simulink model "complex_bouncing"  (Simulink 9.2)
settings: Solver=VariableStepAuto  StartTime=0.0  StopTime=5  FixedStep=1e-3  MaxStep=1e-3  RelTol=1e-6
libraries: simulink x1
settings Model: Creator=jinwooro  LastModifiedBy=jinwooro
settings SolverCC: ZeroCrossAlgorithm=Adaptive
settings DataIOCC: LimitDataPoints=off  SaveFormat=Dataset  SignalLoggingSaveFormat=Dataset
settings OptimizationCC: LifeSpan=auto
settings DebuggingCC: UnderspecifiedInitializationDetection=Simplified  MergeDetectMultiDrivingBlocksExec=error  IgnoredZcDiagnostic=none  FcnCallInpInsideContextMsg=error  StateNameClashWarn=none  SFUnexpectedBacktrackingDiag=error  SFNoUnconditionalDefaultTransitionDiag=error  SFExecutionAtInitializationDiag=warning
settings HardwareCC: ProdBitPerPointer=64  ProdBitPerSizeT=64  ProdBitPerPtrDiffT=64  ProdLargestAtomicFloat=Float  ProdIntDivRoundTo=Zero  ProdEndianess=LittleEndian  ProdWordSize=64  ProdHWDeviceType=Intel->x86-64 (Windows64)
settings ModelReferenceCC: PropagateSignalLabelsOutOfModel=on
settings SFSimCC: SimUseLocalCustomCode=on
settings RTWCC: RTWUseLocalCustomCode=on
settings CodeAppCC: StateflowObjectComments=off
settings GRTTargetCC: TargetLangStandard=C99 (ISO)  GeneratePreprocessorConditionals=Use local settings  CombineOutputUpdateFcns=on  GRTInterface=off
settings ConfigComp: CovMetricSettings=dwe  CovHtmlReporting=off  CovSaveCumulativeToWorkspaceVar=off  CovSaveSingleToWorkspaceVar=off  CovExternalEMLEnable=on

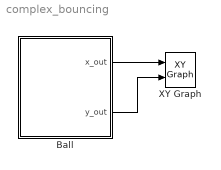
== system complex_bouncing ==
  Ball : Stateflow chart  TreatAsAtomicUnit=on
  XY Graph : simulink/Sinks/XY Graph  xmin=0  xmax=25  ymin=-2  ymax=7  st=-1
  wires:
  Ball/1(x_out) -> XY Graph/1
  Ball/2(y_out) -> XY Graph/2

== stateflow chart Ball ==
  settings: updateMethod=CONTINUOUS
  state BouncingBall
    du:
    x_dot =  vx;
    y_dot = vy;
    vx_dot = 0;
    vy_dot = -9.8;
    x_out = x;
    y_out = y;
  note: vx = ( sin(x) * sin(x) * vx + 2 * cos(x) * vy ) / (1 + cos(x) * cos(x));
      | vy = (2 * cos(x) * vx - sin(x) * sin(x) * vy) / (1 + cos(x) * cos(x));
  note: vx = ((1- 0.8 * sin(x) * sin(x)) * vx + 1.8 * vy * cos(x)) / (1 + cos(x) * cos(x));
      | vy = (1.8 * vx * cos(x) + (-0.8 + sin(x) * sin(x)) * vy) / (1 + cos(x) * cos(x));
  (default) -> BouncingBall : { vx = 4; vy = 3; x = 0; y = 1; }
  BouncingBall -> BouncingBall : [ sin(x) >= y ] {
      | vx = ( sin(x) * sin(x) * vx + 2 * cos(x) * vy ) / (1 + cos(x) * cos(x));
      | vy = (2 * cos(x) * vx - sin(x) * sin(x) * vy) / (1 + cos(x) * cos(x));
      | }
  data: x_out output double; x local double; vx local double; y local double; y_out output double; vy local double
  data x settings: updateMethod=SF_CONTINUOUS_TIME_DATA
  data vx settings: updateMethod=SF_CONTINUOUS_TIME_DATA
  data y settings: updateMethod=SF_CONTINUOUS_TIME_DATA
  data vy settings: updateMethod=SF_CONTINUOUS_TIME_DATA
